simulink model "seconf_task"  (R2022a)
settings: Solver=VariableStepAuto  StartTime=0.0  StopTime=10.0  RelTol=1e-3
libraries: commdigbbndcpm2 x7, commrandsrc3 x1, commutil2 x1
settings Model: Creator=Admin  LastModifiedBy=Admin

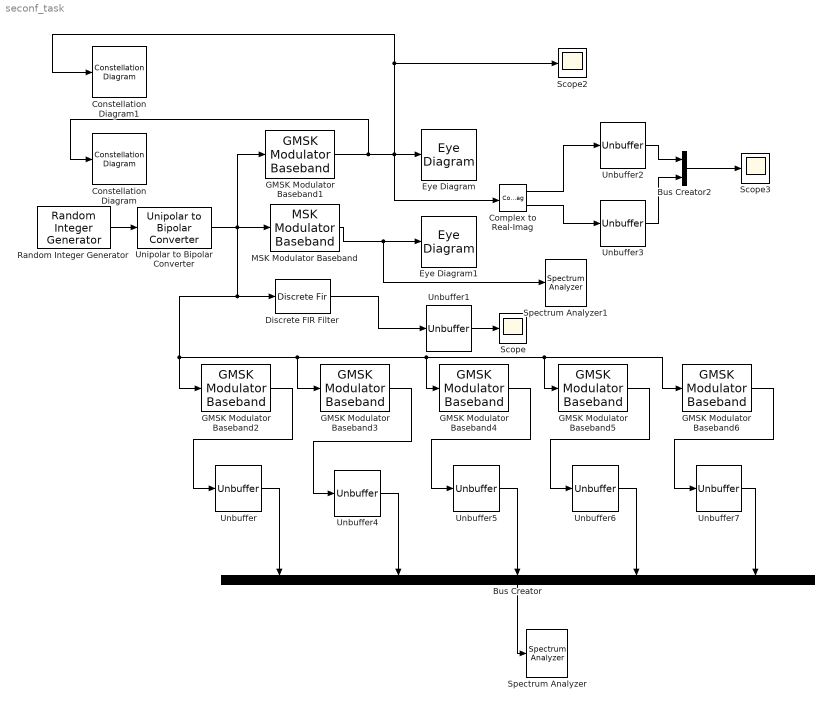
== system seconf_task ==
  Bus Creator : BusCreator  Inputs=5
  Bus Creator2 : BusCreator  Inputs=2
  Complex to Real-Imag : ComplexToRealImag
  Constellation Diagram : ConstellationDiagram  WindowPosition=[382.000000,84.000000,600.000000,600.000000,]  ScopeFrameLocation=window
  Constellation Diagram1 : ConstellationDiagram  WindowPosition=[382.000000,84.000000,600.000000,600.000000,]  ScopeFrameLocation=window
  Discrete FIR Filter : DiscreteFir
  Eye Diagram : EyeDiagram
  Eye Diagram1 : EyeDiagram
  GMSK Modulator Baseband1 : commdigbbndcpm2/GMSK Modulator Baseband  inputType=Integer  BT=.3  pulseLength=4  preHistory=1  phaseOffset=0  samplesPerSymbol=8  RateOptions=Enforce single-rate processing  outDataType=double
      settings: SourceProductBaseCode=CM
  GMSK Modulator Baseband2 : commdigbbndcpm2/GMSK Modulator Baseband  inputType=Integer  BT=1  pulseLength=4  preHistory=1  phaseOffset=0  samplesPerSymbol=8  RateOptions=Enforce single-rate processing  outDataType=double
      settings: SourceProductBaseCode=CM
  GMSK Modulator Baseband3 : commdigbbndcpm2/GMSK Modulator Baseband  inputType=Integer  BT=.7  pulseLength=4  preHistory=1  phaseOffset=0  samplesPerSymbol=8  RateOptions=Enforce single-rate processing  outDataType=double
      settings: SourceProductBaseCode=CM
  GMSK Modulator Baseband4 : commdigbbndcpm2/GMSK Modulator Baseband  inputType=Integer  BT=.5  pulseLength=4  preHistory=1  phaseOffset=0  samplesPerSymbol=8  RateOptions=Enforce single-rate processing  outDataType=double
      settings: SourceProductBaseCode=CM
  GMSK Modulator Baseband5 : commdigbbndcpm2/GMSK Modulator Baseband  inputType=Integer  BT=.3  pulseLength=4  preHistory=1  phaseOffset=0  samplesPerSymbol=8  RateOptions=Enforce single-rate processing  outDataType=double
      settings: SourceProductBaseCode=CM
  GMSK Modulator Baseband6 : commdigbbndcpm2/GMSK Modulator Baseband  inputType=Integer  BT=.3  pulseLength=4  preHistory=1  phaseOffset=0  samplesPerSymbol=8  RateOptions=Enforce single-rate processing  outDataType=double
      settings: SourceProductBaseCode=CM
  MSK Modulator Baseband : commdigbbndcpm2/MSK Modulator Baseband  inputType=Integer  phaseOffset=0  samplesPerSymbol=8  RateOptions=Enforce single-rate processing  outDataType=double
      settings: SourceProductBaseCode=CM
  Random Integer Generator : commrandsrc3/Random Integer Generator  SetSize=8  SeedSource=Auto  Seed=0  SampleTime=1/270000  SamplesPerFrame=1  OutputDataType=uint32  SimulateUsing=Interpreted execution
  Scope : Scope
  Scope2 : Scope
  Scope3 : Scope
  Spectrum Analyzer : SpectrumAnalyzer
  Spectrum Analyzer1 : SpectrumAnalyzer  IsFrequencyInputMode=1
  Unbuffer{,1..7} (8 alike) : Unbuffer
  Unipolar to Bipolar Converter : commutil2/Unipolar to Bipolar Converter  M=2  polarity=Positive  dataType=double
  wires:
  Random Integer Generator/1 -> Unipolar to Bipolar Converter/1
  Unipolar to Bipolar Converter/1 -> MSK Modulator Baseband/1, GMSK Modulator Baseband1/1, GMSK Modulator Baseband3/1, GMSK Modulator Baseband4/1, GMSK Modulator Baseband5/1, GMSK Modulator Baseband6/1, GMSK Modulator Baseband2/1, Discrete FIR Filter/1
  GMSK Modulator Baseband2/1 -> Unbuffer/1
  Unbuffer/1 -> Bus Creator/1
  Bus Creator/1 -> Spectrum Analyzer/1
  GMSK Modulator Baseband1/1 -> Constellation Diagram/1, Complex to Real-Imag/1, Constellation Diagram1/1, Scope2/1, Eye Diagram/1
  MSK Modulator Baseband/1 -> Spectrum Analyzer1/1, Eye Diagram1/1
  Discrete FIR Filter/1 -> Unbuffer1/1
  Unbuffer1/1 -> Scope/1
  Complex to Real-Imag/1 -> Unbuffer2/1
  Complex to Real-Imag/2 -> Unbuffer3/1
  Unbuffer3/1 -> Bus Creator2/2
  Unbuffer2/1 -> Bus Creator2/1
  Bus Creator2/1 -> Scope3/1
  GMSK Modulator Baseband3/1 -> Unbuffer4/1
  Unbuffer4/1 -> Bus Creator/2
  GMSK Modulator Baseband4/1 -> Unbuffer5/1
  Unbuffer5/1 -> Bus Creator/3
  GMSK Modulator Baseband5/1 -> Unbuffer6/1
  Unbuffer6/1 -> Bus Creator/4
  GMSK Modulator Baseband6/1 -> Unbuffer7/1
  Unbuffer7/1 -> Bus Creator/5
